simulink library "thermochemical"  (R2017b)
settings: Solver=VariableStepAuto  StartTime=0.0  StopTime=10.0  RelTol=1e-3
values from neighbouring files (symbols this model uses):
  c = conversion_factors()    [blk_clausius_clapeyron.m]    (also in blk_clausius_clapeyron_no_popup.m; blk_cold_room_closed_dry_air.m; blk_reactor_BaCl2_NH3_no_walls.m; blk_reactor_BaCl2_NH3_no_walls_state_space.m)
  cp = metal.cp    [blk_wall_simple.m]    (also in get_metal_properties.m = 390)
  fluid = get_param(blk,'fluid')    [blk_thermodynamic_properties_nonsaturated.m]    (also in blk_thermodynamic_properties_nonsaturated_interpreted.m; blk_thermodynamic_properties_saturated.m; blk_thermodynamic_properties_saturated_interpreted.m; blk_thermodynamic_properties_saturated_mix.m)
  gas = get_material_properties(x.gasName)    [blk_reactor_BaCl2_NH3_cylindrical_no_walls_fun1.m]
  h = get_param(gcb,'ObjectParameters')    [get_param_eval.m]
  rho = metal.rho    [blk_wall_simple.m]    (also in get_metal_properties.m = 8940)
  s = solve(eq,dx,'ReturnConditions',true)    [LMTD_inv.m]    (also in blk_wall_simple.m = get_param_eval(blk,'s'))
  u_gas_at_T_ref = -R * T_ref    [blk_reactor_BaCl2_NH3_no_walls.m]    (also in blk_reactor_BaCl2_NH3_no_walls_state_space.m)
undefined symbols (not defined in the file or in its folder): b_motor, BaCl2, beta, CoolProp, cP_binder, cP_gas, cP_s0, cv, dh_r_0, ENG, heat_exchanger_epsilonNTU_inv_simulink, heat_exchanger_epsilonNTU_simulink, J_motor, K_cin, kappa, Km_motor, La_motor, lookup2D_BreakPoint2, M_binder, N_binder, N_gas_free_volume_init, N_salt, NH3, nh3_v3, nu, P, phase, PID_D_motor, PID_I_motor, PID_P_motor, Ra_motor, Reactor_phase, T, T1, T2, T_init, Tr_init, Tr_ref, U_binder_at_Tr_ref, U_salt_at_X0_Tr_ref, Ur_init, V_void, Valve_regime, Vmax_motor, w_init_motor, X_init
libraries: thermochemical x247, simulink x54, dspsigops x3
(part 7 of 12)

== system thermochemical/Reactors/Reactor, BaCl2//NH3, state-space form, [Tr, Ng, X] as state variables, no algebraic loops, real gas in void volume, ideal gas in salt/Reactor, BaCl2, cylindrical, finned tube, state-space form, [Tr, Ng, X] as state variables, no algebraic loops, real gas in void volume, ideal gas in salt ==
  In3 : Inport
  In1 : Inport  Port=2
  In2 : Inport  Port=3
  In4 : Inport  Port=4
  Display4 : Display
  Gain : Gain  Gain=-1
  "Reactor, BaCl2/NH3, cylindrical, no walls, state-space form, [Tr, Ng, X] as state variables, no algebraic loops, real gas in void volume, ideal gas in salt" : thermochemical/Reactors/Reactor, BaCl2//NH3, state-space form, [Tr, Ng, X] as state variables, no algebraic loops, real gas in void volume, ideal gas in salt/Reactor, BaCl2//NH3, cylindrical, no walls, state-space form, [Tr, Ng, X] as state variables, no algebraic loops, real gas in void volume, ideal gas in salt  pairName=Barium chloride/Ammonia (BaCl2/NH3)  gasName=Ammonia gas (NH3)  binderName=ENG  tao_salt=0.75  rho_composite=300  K_cin=1e-3  fluid=nh3_v3  Lr=1.5  Lr_total=1.6  Dr=0.11  Ddiff=0.018  Tr_init=300  X_init=0.1  Vr_L=15.2053  m_composite_kg=4.162  m_salt_kg=3.1215  m_binder_kg=1.0405  m_gas_when_reactor_fully_charged_kg=2.0423  kWh_cold=0.77838  N_salt=14.9906  N_binder=86.6307  V_void=0.001332  N_gas_free_volume_init=0.16063
      settings: SourceProductName=@ Thermochemical
  "Wall, tube with/without fins" : thermochemical/Walls/Wall, tube with//without fins  L_m=1.6  OD_mm=114  e_mm=2  material_tube=Stainless steel AISI316  cp_tube=490.8  rho_tube=8023  height_fin_mm=0  thickness_fin_mm=0  pitch_fin_mm=0  material_fin=Steel  cp_fin=464.5  rho_fin=7847  lambda_fin=64.65  Tinit=300  mass_tube=4.5571  mass_fin=0  mass_total=4.5571  s_inner=0.56297  s_outer=0.57303
      settings: SourceProductName=@ Thermochemical
  composite-wall contact heat transfer coefficient (W/m2/K) : Constant  Value=300
  Out3 : Outport
  Out2 : Outport  Port=2
  Out4 : Outport  Port=3
  Out1 : Outport  Port=4
  Out5 : Outport  Port=5
  Out6 : Outport  Port=6
  Out7 : Outport  Port=7
  Out8 : Outport  Port=8
  wires:
  In4/1 -> "Reactor, BaCl2/NH3, cylindrical, no walls, state-space form, [Tr, Ng, X] as state variables, no algebraic loops, real gas in void volume, ideal gas in salt"/2  "enthalpy in (J/mol) (only needed if dn/dt gas > 0)"
  In2/1 -> "Reactor, BaCl2/NH3, cylindrical, no walls, state-space form, [Tr, Ng, X] as state variables, no algebraic loops, real gas in void volume, ideal gas in salt"/1  "dn/dt gas (mol/sec) > 0: gas in   < 0: gas out"
  "Wall, tube with/without fins"/1 -> Out3/1  "T wall (K)"
  "Reactor, BaCl2/NH3, cylindrical, no walls, state-space form, [Tr, Ng, X] as state variables, no algebraic loops, real gas in void volume, ideal gas in salt"/2 -> Out4/1  "Pr (bar)"
  "Reactor, BaCl2/NH3, cylindrical, no walls, state-space form, [Tr, Ng, X] as state variables, no algebraic loops, real gas in void volume, ideal gas in salt"/5 -> Out6/1  "X (0..1)"
  In1/1 -> "Wall, tube with/without fins"/2  "h outer (W/m2/K)"
  "Wall, tube with/without fins"/3 -> Out8/1  "Q wall → outer (W)"
  In3/1 -> "Wall, tube with/without fins"/1  "T outer (K)"
  "Reactor, BaCl2/NH3, cylindrical, no walls, state-space form, [Tr, Ng, X] as state variables, no algebraic loops, real gas in void volume, ideal gas in salt"/3 -> Out1/1  "h gas (void space) (J/mol)"
  composite-wall contact heat transfer coefficient (W/m2/K)/1 -> "Wall, tube with/without fins"/4
  "Wall, tube with/without fins"/2 -> Out7/1, Gain/1  "Q inner → wall (W)"
  "Reactor, BaCl2/NH3, cylindrical, no walls, state-space form, [Tr, Ng, X] as state variables, no algebraic loops, real gas in void volume, ideal gas in salt"/4 -> Out5/1  "Reaction phase"
  "Reactor, BaCl2/NH3, cylindrical, no walls, state-space form, [Tr, Ng, X] as state variables, no algebraic loops, real gas in void volume, ideal gas in salt"/1 -> "Wall, tube with/without fins"/3, Out2/1  "Tr (K)"
  "Wall, tube with/without fins"/4 -> Display4/1
  Gain/1 -> "Reactor, BaCl2/NH3, cylindrical, no walls, state-space form, [Tr, Ng, X] as state variables, no algebraic loops, real gas in void volume, ideal gas in salt"/3

== system thermochemical/Reactors/Reactor, BaCl2//NH3, state-space form, [Tr, Ng, X] as state variables, no algebraic loops, real gas in void volume, ideal gas in salt/Reactor, BaCl2//NH3, cylindrical, no walls, state-space form, [Tr, Ng, X] as state variables, no algebraic loops, real gas in void volume, ideal gas in salt ==
  In3 : Inport
  In2 : Inport  Port=2
  In4 : Inport  Port=3
  "Reactor, BaCl2/NH3, no walls, state-space form, [Tr, Ng, X] as state variables, no algebraic loops, real gas in void volume, ideal gas in salt" : thermochemical/Reactors/Reactor, BaCl2//NH3, state-space form, [Tr, Ng, X] as state variables, no algebraic loops, real gas in void volume, ideal gas in salt/Reactor, BaCl2//NH3, no walls, state-space form, [Tr, Ng, X] as state variables, no algebraic loops, real gas in void volume, ideal gas in salt  pairName=Barium chloride/Ammonia (BaCl2/NH3)  gasName=Ammonia gas (NH3)  binderName=ENG  N_salt=N_salt  N_binder=N_binder  K_cin=K_cin  V_void=V_void  fluid=fluid  Tr_init=Tr_init  X_init=X_init  N_gas_free_volume_init=N_gas_free_volume_init  m_composite_kg=4.1639  m_salt_kg=3.1235  m_binder_kg=1.0405  m_gas_when_reactor_fully_charged=2.0436  T_ref=300  u_gas_at_T_ref=0  U_binder_at_T_ref=0  U_salt_at_X0_T_ref=0  R=8.3145  cP_gas=42.5775  cV_gas=29.4370  nu=8  cP_s0=75.1  dh_r_0=38250  M_binder=0.012011  cP_binder=714.36  P_dead_zone=0.0001  dn_dead_zone=0.0001
      settings: SourceProductName=@ Thermochemical
  Out2 : Outport
  Out4 : Outport  Port=2
  Out3 : Outport  Port=3
  Out5 : Outport  Port=4
  Out1 : Outport  Port=5
  wires:
  In3/1 -> "Reactor, BaCl2/NH3, no walls, state-space form, [Tr, Ng, X] as state variables, no algebraic loops, real gas in void volume, ideal gas in salt"/1  "dn/dt gas (mol/sec) > 0: gas in   < 0: gas out"
  In2/1 -> "Reactor, BaCl2/NH3, no walls, state-space form, [Tr, Ng, X] as state variables, no algebraic loops, real gas in void volume, ideal gas in salt"/2  "enthalpy in (J/mol) (only needed if dn/dt gas > 0)"
  In4/1 -> "Reactor, BaCl2/NH3, no walls, state-space form, [Tr, Ng, X] as state variables, no algebraic loops, real gas in void volume, ideal gas in salt"/3  "q out → in (W)"
  "Reactor, BaCl2/NH3, no walls, state-space form, [Tr, Ng, X] as state variables, no algebraic loops, real gas in void volume, ideal gas in salt"/5 -> Out1/1  "X (0..1)"
  "Reactor, BaCl2/NH3, no walls, state-space form, [Tr, Ng, X] as state variables, no algebraic loops, real gas in void volume, ideal gas in salt"/4 -> Out5/1  "Reaction phase"
  "Reactor, BaCl2/NH3, no walls, state-space form, [Tr, Ng, X] as state variables, no algebraic loops, real gas in void volume, ideal gas in salt"/3 -> Out3/1  "h gas (void space) (J/mol)"
  "Reactor, BaCl2/NH3, no walls, state-space form, [Tr, Ng, X] as state variables, no algebraic loops, real gas in void volume, ideal gas in salt"/2 -> Out4/1  "Pr (bar)"
  "Reactor, BaCl2/NH3, no walls, state-space form, [Tr, Ng, X] as state variables, no algebraic loops, real gas in void volume, ideal gas in salt"/1 -> Out2/1  "Tr (K)"

== system thermochemical/Reactors/Reactor, BaCl2//NH3, state-space form, [Tr, Ng, X] as state variables, no algebraic loops, real gas in void volume, ideal gas in salt/Reactor, BaCl2//NH3, no walls, state-space form, [Tr, Ng, X] as state variables, no algebraic loops, real gas in void volume, ideal gas in salt ==
  In3 : Inport
  In2 : Inport  Port=2
  In4 : Inport  Port=3
  "Reactor, no walls, state space form" : Subsystem
  Out2 : Outport
  Out1 : Outport  Port=2
  Out5 : Outport  Port=3
  Out3 : Outport  Port=4
  Out4 : Outport  Port=5
  wires:
  In3/1 -> "Reactor, no walls, state space form"/2(enthalpy_in (J/mol) (only if dn_gas > 0))  "dn/dt gas (mol/sec) > 0: gas in   < 0: gas out"
  In2/1 -> "Reactor, no walls, state space form"/3(In3)  "enthalpy in (J/mol) (only needed if dn/dt gas > 0)"
  In4/1 -> "Reactor, no walls, state space form"/1(q reactor → wall (W))  "q out → in (W)"
  "Reactor, no walls, state space form"/2(Reactor phase) -> Out1/1  "Pr (bar)"
  "Reactor, no walls, state space form"/4(T_reactor (K)) -> Out5/1  "h gas void space (J/mol)"
  "Reactor, no walls, state space form"/5(h_reactor_free_volume (J/mol)) -> Out3/1  "Reaction phase"
  "Reactor, no walls, state space form"/3(P_reactor (bar)) -> Out4/1  "X (0..1)"
  "Reactor, no walls, state space form"/1(X (0..1)) -> Out2/1  "Tr (K)"

== system thermochemical/Reactors/Reactor, BaCl2//NH3, state-space form, [Tr, Ng, X] as state variables, no algebraic loops, real gas in void volume, real gas in salt/Reactor, BaCl2, cylindrical, finned tube, state-space form, [Tr, Ng, X] as state variables, no algebraic loops, real gas in void volume, real gas in salt ==
  In3 : Inport
  In1 : Inport  Port=2
  In2 : Inport  Port=3
  In4 : Inport  Port=4
  Display4 : Display
  Gain : Gain  Gain=-1
  "Reactor, BaCl2/NH3, cylindrical, no walls, state-space form, [Tr, Ng, X] as state variables, no algebraic loops, real gas in void volume, real gas in salt" : thermochemical/Reactors/Reactor, BaCl2//NH3, state-space form, [Tr, Ng, X] as state variables, no algebraic loops, real gas in void volume, real gas in salt/Reactor, BaCl2//NH3, cylindrical, no walls, state-space form, [Tr, Ng, X] as state variables, no algebraic loops, real gas in void volume, real gas in salt  pairName=Barium chloride/Ammonia (BaCl2/NH3)  gasName=Ammonia gas (NH3)  binderName=ENG  tao_salt=0.75  rho_composite=300  K_cin=1e-3  fluid=nh3_v3  Lr=1.5  Lr_total=1.6  Dr=0.11  Ddiff=0.018  Tr_init=300  X_init=0.1  Vr_L=15.2053  m_composite_kg=4.162  m_salt_kg=3.1215  m_binder_kg=1.0405  m_gas_when_reactor_fully_charged_kg=2.0423  kWh_cold=0.77838  N_salt=14.9906  N_binder=86.6307  V_void=0.001332  N_gas_free_volume_init=0.16063
      settings: SourceProductName=@ Thermochemical
  "Wall, tube with/without fins" : thermochemical/Walls/Wall, tube with//without fins  L_m=1.6  OD_mm=114  e_mm=2  material_tube=Stainless steel AISI316  cp_tube=490.8  rho_tube=8023  height_fin_mm=0  thickness_fin_mm=0  pitch_fin_mm=0  material_fin=Steel  cp_fin=464.5  rho_fin=7847  lambda_fin=64.65  Tinit=300  mass_tube=9.0335  mass_fin=0  mass_total=9.0335  s_inner=0.55292  s_outer=0.57303
      settings: SourceProductName=@ Thermochemical
  composite-wall contact heat transfer coefficient (W/m2/K) : Constant  Value=300
  Out3 : Outport
  Out2 : Outport  Port=2
  Out4 : Outport  Port=3
  Out1 : Outport  Port=4
  Out5 : Outport  Port=5
  Out6 : Outport  Port=6
  Out7 : Outport  Port=7
  Out8 : Outport  Port=8
  wires:
  In4/1 -> "Reactor, BaCl2/NH3, cylindrical, no walls, state-space form, [Tr, Ng, X] as state variables, no algebraic loops, real gas in void volume, real gas in salt"/2  "enthalpy in (J/mol) (only needed if dn/dt gas > 0)"
  In2/1 -> "Reactor, BaCl2/NH3, cylindrical, no walls, state-space form, [Tr, Ng, X] as state variables, no algebraic loops, real gas in void volume, real gas in salt"/1  "dn/dt gas (mol/sec) > 0: gas in   < 0: gas out"
  "Wall, tube with/without fins"/1 -> Out3/1  "T wall (K)"
  "Reactor, BaCl2/NH3, cylindrical, no walls, state-space form, [Tr, Ng, X] as state variables, no algebraic loops, real gas in void volume, real gas in salt"/2 -> Out4/1  "Pr (bar)"
  "Reactor, BaCl2/NH3, cylindrical, no walls, state-space form, [Tr, Ng, X] as state variables, no algebraic loops, real gas in void volume, real gas in salt"/5 -> Out6/1  "X (0..1)"
  In1/1 -> "Wall, tube with/without fins"/2  "h outer (W/m2/K)"
  "Wall, tube with/without fins"/3 -> Out8/1  "Q wall → outer (W)"
  In3/1 -> "Wall, tube with/without fins"/1  "T outer (K)"
  "Reactor, BaCl2/NH3, cylindrical, no walls, state-space form, [Tr, Ng, X] as state variables, no algebraic loops, real gas in void volume, real gas in salt"/3 -> Out1/1  "h gas (void space) (J/mol)"
  composite-wall contact heat transfer coefficient (W/m2/K)/1 -> "Wall, tube with/without fins"/4
  "Wall, tube with/without fins"/2 -> Out7/1, Gain/1  "Q inner → wall (W)"
  "Reactor, BaCl2/NH3, cylindrical, no walls, state-space form, [Tr, Ng, X] as state variables, no algebraic loops, real gas in void volume, real gas in salt"/4 -> Out5/1  "Reaction phase"
  "Reactor, BaCl2/NH3, cylindrical, no walls, state-space form, [Tr, Ng, X] as state variables, no algebraic loops, real gas in void volume, real gas in salt"/1 -> "Wall, tube with/without fins"/3, Out2/1  "Tr (K)"
  "Wall, tube with/without fins"/4 -> Display4/1
  Gain/1 -> "Reactor, BaCl2/NH3, cylindrical, no walls, state-space form, [Tr, Ng, X] as state variables, no algebraic loops, real gas in void volume, real gas in salt"/3

== system thermochemical/Reactors/Reactor, BaCl2//NH3, state-space form, [Tr, Ng, X] as state variables, no algebraic loops, real gas in void volume, real gas in salt/Reactor, BaCl2//NH3, cylindrical, no walls, state-space form, [Tr, Ng, X] as state variables, no algebraic loops, real gas in void volume, real gas in salt ==
  In3 : Inport
  In2 : Inport  Port=2
  In4 : Inport  Port=3
  "Reactor, BaCl2/NH3, no walls, state-space form, [Tr, Ng, X] as state variables, no algebraic loops, real gas in void volume, real gas in salt" : thermochemical/Reactors/Reactor, BaCl2//NH3, state-space form, [Tr, Ng, X] as state variables, no algebraic loops, real gas in void volume, real gas in salt/Reactor, BaCl2//NH3, no walls, state-space form, [Tr, Ng, X] as state variables, no algebraic loops, real gas in void volume, real gas in salt  pairName=Barium chloride/Ammonia (BaCl2/NH3)  gasName=Ammonia gas (NH3)  binderName=ENG  N_salt=N_salt  N_binder=N_binder  K_cin=K_cin  V_void=V_void  fluid=fluid  Tr_init=Tr_init  X_init=X_init  N_gas_free_volume_init=N_gas_free_volume_init  m_composite_kg=4.1639  m_salt_kg=3.1235  m_binder_kg=1.0405  m_gas_when_reactor_fully_charged=2.0436  T_ref=300  u_gas_at_T_ref=0  U_binder_at_T_ref=0  U_salt_at_X0_T_ref=0  R=8.3145  cP_gas=42.5775  cV_gas=29.4370  nu=8  cP_s0=75.1  dh_r_0=38250  M_binder=0.012011  cP_binder=714.36  P_dead_zone=0.0001  dn_dead_zone=0.0001
      settings: SourceProductName=@ Thermochemical
  Out2 : Outport
  Out4 : Outport  Port=2
  Out3 : Outport  Port=3
  Out5 : Outport  Port=4
  Out1 : Outport  Port=5
  wires:
  In3/1 -> "Reactor, BaCl2/NH3, no walls, state-space form, [Tr, Ng, X] as state variables, no algebraic loops, real gas in void volume, real gas in salt"/1  "dn/dt gas (mol/sec) > 0: gas in   < 0: gas out"
  In2/1 -> "Reactor, BaCl2/NH3, no walls, state-space form, [Tr, Ng, X] as state variables, no algebraic loops, real gas in void volume, real gas in salt"/2  "enthalpy in (J/mol) (only needed if dn/dt gas > 0)"
  In4/1 -> "Reactor, BaCl2/NH3, no walls, state-space form, [Tr, Ng, X] as state variables, no algebraic loops, real gas in void volume, real gas in salt"/3  "q out → in (W)"
  "Reactor, BaCl2/NH3, no walls, state-space form, [Tr, Ng, X] as state variables, no algebraic loops, real gas in void volume, real gas in salt"/5 -> Out1/1  "X (0..1)"
  "Reactor, BaCl2/NH3, no walls, state-space form, [Tr, Ng, X] as state variables, no algebraic loops, real gas in void volume, real gas in salt"/4 -> Out5/1  "Reaction phase"
  "Reactor, BaCl2/NH3, no walls, state-space form, [Tr, Ng, X] as state variables, no algebraic loops, real gas in void volume, real gas in salt"/3 -> Out3/1  "h gas (void space) (J/mol)"
  "Reactor, BaCl2/NH3, no walls, state-space form, [Tr, Ng, X] as state variables, no algebraic loops, real gas in void volume, real gas in salt"/2 -> Out4/1  "Pr (bar)"
  "Reactor, BaCl2/NH3, no walls, state-space form, [Tr, Ng, X] as state variables, no algebraic loops, real gas in void volume, real gas in salt"/1 -> Out2/1  "Tr (K)"

== system thermochemical/Reactors/Reactor, BaCl2//NH3, state-space form, [Tr, Ng, X] as state variables, no algebraic loops, real gas in void volume, real gas in salt/Reactor, BaCl2//NH3, no walls, state-space form, [Tr, Ng, X] as state variables, no algebraic loops, real gas in void volume, real gas in salt ==
  In3 : Inport
  In2 : Inport  Port=2
  In4 : Inport  Port=3
  "Reactor, no walls, state space form" : Subsystem
  Out2 : Outport
  Out1 : Outport  Port=2
  Out5 : Outport  Port=3
  Out3 : Outport  Port=4
  Out4 : Outport  Port=5
  wires:
  "Reactor, no walls, state space form"/1(X (0..1)) -> Out2/1  "Tr (K)"
  "Reactor, no walls, state space form"/3(P_reactor (bar)) -> Out4/1  "X (0..1)"
  "Reactor, no walls, state space form"/5(h_reactor_free_volume (J/mol)) -> Out3/1  "Reaction phase"
  "Reactor, no walls, state space form"/4(T_reactor (K)) -> Out5/1  "h gas void space (J/mol)"
  "Reactor, no walls, state space form"/2(Reactor phase) -> Out1/1  "Pr (bar)"
  In4/1 -> "Reactor, no walls, state space form"/1(q reactor → wall (W))  "q out → in (W)"
  In2/1 -> "Reactor, no walls, state space form"/3(In3)  "enthalpy in (J/mol) (only needed if dn/dt gas > 0)"
  In3/1 -> "Reactor, no walls, state space form"/2(enthalpy_in (J/mol) (only if dn_gas > 0))  "dn/dt gas (mol/sec) > 0: gas in   < 0: gas out"

== system thermochemical/Reactors/Reactor, BaCl2//NH3, state-space form, [Ur, Ng, X] as state variables, no algebraic loops, ideal gas in void volume, ideal gas in salt/Reactor, BaCl2, cylindrical, finned tube, state-space form, [Ur, Ng, X] as state variables, no algebraic loops, ideal gas in void volume, ideal gas in salt ==
  In3 : Inport
  In1 : Inport  Port=2
  In2 : Inport  Port=3
  In4 : Inport  Port=4
  Display4 : Display
  Gain : Gain  Gain=-1
  "Reactor, BaCl2/NH3, cylindrical, no walls, state-space form, [Ur, Ng, X] as state variables, no algebraic loops, ideal gas in void volume, ideal gas in salt" : thermochemical/Reactors/Reactor, BaCl2//NH3, state-space form, [Ur, Ng, X] as state variables, no algebraic loops, ideal gas in void volume, ideal gas in salt/Reactor, BaCl2//NH3, cylindrical, no walls, state-space form, [Ur, Ng, X] as state variables, no algebraic loops, ideal gas in void volume, ideal gas in salt  pairName=Barium chloride/Ammonia (BaCl2/NH3)  gasName=Ammonia gas (NH3)  binderName=ENG  tao_salt=0.75  rho_composite=300  K_cin=1e-3  fluid=nh3_v3  Lr=1.5  Lr_total=1.6  Dr=0.11  Ddiff=0.018  Tr_init=300  X_init=0.1  Vr_L=15.2053  m_composite_kg=4.162  m_salt_kg=3.1215  m_binder_kg=1.0405  m_gas_when_reactor_fully_charged_kg=2.0423  kWh_cold=0.77838  N_salt=14.9906  N_binder=86.6307  V_void=0.001332  N_gas_free_volume_init=0.16063
      settings: SourceProductName=@ Thermochemical
  "Wall, tube with/without fins" : thermochemical/Walls/Wall, tube with//without fins  L_m=1.6  OD_mm=114  e_mm=2  material_tube=Stainless steel AISI316  cp_tube=490.8  rho_tube=8023  height_fin_mm=0  thickness_fin_mm=0  pitch_fin_mm=0  material_fin=Steel  cp_fin=464.5  rho_fin=7847  lambda_fin=64.65  Tinit=300  mass_tube=4.5571  mass_fin=0  mass_total=4.5571  s_inner=0.56297  s_outer=0.57303
      settings: SourceProductName=@ Thermochemical
  composite-wall contact heat transfer coefficient (W/m2/K) : Constant  Value=300
  Out3 : Outport
  Out2 : Outport  Port=2
  Out4 : Outport  Port=3
  Out1 : Outport  Port=4
  Out5 : Outport  Port=5
  Out6 : Outport  Port=6
  Out7 : Outport  Port=7
  Out8 : Outport  Port=8
  wires:
  In4/1 -> "Reactor, BaCl2/NH3, cylindrical, no walls, state-space form, [Ur, Ng, X] as state variables, no algebraic loops, ideal gas in void volume, ideal gas in salt"/2  "enthalpy in (J/mol) (only needed if dn/dt gas > 0)"
  In2/1 -> "Reactor, BaCl2/NH3, cylindrical, no walls, state-space form, [Ur, Ng, X] as state variables, no algebraic loops, ideal gas in void volume, ideal gas in salt"/1  "dn/dt gas (mol/sec) > 0: gas in   < 0: gas out"
  "Wall, tube with/without fins"/1 -> Out3/1  "T wall (K)"
  "Reactor, BaCl2/NH3, cylindrical, no walls, state-space form, [Ur, Ng, X] as state variables, no algebraic loops, ideal gas in void volume, ideal gas in salt"/2 -> Out4/1  "Pr (bar)"
  "Reactor, BaCl2/NH3, cylindrical, no walls, state-space form, [Ur, Ng, X] as state variables, no algebraic loops, ideal gas in void volume, ideal gas in salt"/5 -> Out6/1  "X (0..1)"
  In1/1 -> "Wall, tube with/without fins"/2  "h outer (W/m2/K)"
  "Wall, tube with/without fins"/3 -> Out8/1  "Q wall → outer (W)"
  In3/1 -> "Wall, tube with/without fins"/1  "T outer (K)"
  "Reactor, BaCl2/NH3, cylindrical, no walls, state-space form, [Ur, Ng, X] as state variables, no algebraic loops, ideal gas in void volume, ideal gas in salt"/3 -> Out1/1  "h gas (void space) (J/mol)"
  composite-wall contact heat transfer coefficient (W/m2/K)/1 -> "Wall, tube with/without fins"/4
  "Wall, tube with/without fins"/2 -> Out7/1, Gain/1  "Q inner → wall (W)"
  "Reactor, BaCl2/NH3, cylindrical, no walls, state-space form, [Ur, Ng, X] as state variables, no algebraic loops, ideal gas in void volume, ideal gas in salt"/4 -> Out5/1  "Reaction phase"
  "Reactor, BaCl2/NH3, cylindrical, no walls, state-space form, [Ur, Ng, X] as state variables, no algebraic loops, ideal gas in void volume, ideal gas in salt"/1 -> "Wall, tube with/without fins"/3, Out2/1  "Tr (K)"
  "Wall, tube with/without fins"/4 -> Display4/1
  Gain/1 -> "Reactor, BaCl2/NH3, cylindrical, no walls, state-space form, [Ur, Ng, X] as state variables, no algebraic loops, ideal gas in void volume, ideal gas in salt"/3

== system thermochemical/Reactors/Reactor, BaCl2//NH3, state-space form, [Ur, Ng, X] as state variables, no algebraic loops, ideal gas in void volume, ideal gas in salt/Reactor, BaCl2//NH3, cylindrical, no walls, state-space form, [Ur, Ng, X] as state variables, no algebraic loops, ideal gas in void volume, ideal gas in salt ==
  In3 : Inport
  In2 : Inport  Port=2
  In4 : Inport  Port=3
  "Reactor, BaCl2/NH3, no walls, state-space form, [Ur, Ng, X] as state variables, no algebraic loops, ideal gas in void volume, ideal gas in salt" : thermochemical/Reactors/Reactor, BaCl2//NH3, state-space form, [Ur, Ng, X] as state variables, no algebraic loops, ideal gas in void volume, ideal gas in salt/Reactor, BaCl2//NH3, no walls, state-space form, [Ur, Ng, X] as state variables, no algebraic loops, ideal gas in void volume, ideal gas in salt  pairName=Barium chloride/Ammonia (BaCl2/NH3)  gasName=Ammonia gas (NH3)  binderName=ENG  N_salt=N_salt  N_binder=N_binder  K_cin=K_cin  V_void=V_void  Tr_init=Tr_init  X_init=X_init  N_gas_free_volume_init=N_gas_free_volume_init  T_ref=239.8236  u_gas_at_T_ref=-1994.0066  U_binder_at_T_ref=0  U_salt_at_X0_T_ref=0  R=8.3145  cP_gas=42.5775  nu=8  cP_s0=75.1  dh_r_0=38250  M_binder=0.012011  cP_binder=714.36  P_dead_zone=0.0001  dn_dead_zone=0.0001
      settings: SourceProductName=@ Thermochemical
  Out2 : Outport
  Out4 : Outport  Port=2
  Out3 : Outport  Port=3
  Out5 : Outport  Port=4
  Out1 : Outport  Port=5
  wires:
  In3/1 -> "Reactor, BaCl2/NH3, no walls, state-space form, [Ur, Ng, X] as state variables, no algebraic loops, ideal gas in void volume, ideal gas in salt"/1  "dn/dt gas (mol/sec) > 0: gas in   < 0: gas out"
  In2/1 -> "Reactor, BaCl2/NH3, no walls, state-space form, [Ur, Ng, X] as state variables, no algebraic loops, ideal gas in void volume, ideal gas in salt"/2  "enthalpy in (J/mol) (only needed if dn/dt gas > 0)"
  In4/1 -> "Reactor, BaCl2/NH3, no walls, state-space form, [Ur, Ng, X] as state variables, no algebraic loops, ideal gas in void volume, ideal gas in salt"/3  "q out → in (W)"
  "Reactor, BaCl2/NH3, no walls, state-space form, [Ur, Ng, X] as state variables, no algebraic loops, ideal gas in void volume, ideal gas in salt"/5 -> Out1/1  "X (0..1)"
  "Reactor, BaCl2/NH3, no walls, state-space form, [Ur, Ng, X] as state variables, no algebraic loops, ideal gas in void volume, ideal gas in salt"/4 -> Out5/1  "Reaction phase"
  "Reactor, BaCl2/NH3, no walls, state-space form, [Ur, Ng, X] as state variables, no algebraic loops, ideal gas in void volume, ideal gas in salt"/3 -> Out3/1  "h gas (void space) (J/mol)"
  "Reactor, BaCl2/NH3, no walls, state-space form, [Ur, Ng, X] as state variables, no algebraic loops, ideal gas in void volume, ideal gas in salt"/2 -> Out4/1  "Pr (bar)"
  "Reactor, BaCl2/NH3, no walls, state-space form, [Ur, Ng, X] as state variables, no algebraic loops, ideal gas in void volume, ideal gas in salt"/1 -> Out2/1  "Tr (K)"

== system thermochemical/Reactors/Reactor, BaCl2//NH3, state-space form, [Ur, Ng, X] as state variables, no algebraic loops, ideal gas in void volume, ideal gas in salt/Reactor, BaCl2//NH3, no walls, state-space form, [Ur, Ng, X] as state variables, no algebraic loops, ideal gas in void volume, ideal gas in salt ==
  In3 : Inport
  In2 : Inport  Port=2
  In4 : Inport  Port=3
  "Reactor, no walls, state space form" : Subsystem
  Out2 : Outport
  Out1 : Outport  Port=2
  Out5 : Outport  Port=3
  Out3 : Outport  Port=4
  Out4 : Outport  Port=5
  wires:
  "Reactor, no walls, state space form"/1(X (0..1)) -> Out2/1  "Tr (K)"
  "Reactor, no walls, state space form"/3(P_reactor (bar)) -> Out4/1  "X (0..1)"
  "Reactor, no walls, state space form"/5(h_reactor_free_volume (J/mol)) -> Out3/1  "Reaction phase"
  "Reactor, no walls, state space form"/4(T_reactor (K)) -> Out5/1  "h gas void space (J/mol)"
  "Reactor, no walls, state space form"/2(Reactor phase) -> Out1/1  "Pr (bar)"
  In4/1 -> "Reactor, no walls, state space form"/1(q reactor → wall (W))  "q out → in (W)"
  In2/1 -> "Reactor, no walls, state space form"/3(In3)  "enthalpy in (J/mol) (only needed if dn/dt gas > 0)"
  In3/1 -> "Reactor, no walls, state space form"/2(enthalpy_in (J/mol) (only if dn_gas > 0))  "dn/dt gas (mol/sec) > 0: gas in   < 0: gas out"

== system thermochemical/Reactors/Reactor, BaCl2//NH3, with algebraic loops, ideal gas in void volume, ideal gas in salt/Reactor, BaCl2, cylindrical, finned tube, with algebraic loops, ideal gas in void volume, ideal gas in salt ==
  In3 : Inport
  In1 : Inport  Port=2
  In2 : Inport  Port=3
  In4 : Inport  Port=4
  Display4 : Display
  Gain : Gain  Gain=-1
  "Reactor, BaCl2/NH3, cylindrical, no walls, with algebraic loops, ideal gas in void volume, ideal gas in salt" : thermochemical/Reactors/Reactor, BaCl2//NH3, with algebraic loops, ideal gas in void volume, ideal gas in salt/Reactor, BaCl2//NH3, cylindrical, no walls, with algebraic loops, ideal gas in void volume, ideal gas in salt  pairName=Barium chloride/Ammonia (BaCl2/NH3)  gasName=Ammonia gas (NH3)  binderName=ENG  tao_salt=0.75  rho_composite=300  K_cin=1e-3  fluid=nh3_v3  Lr=1.5  Lr_total=1.6  Dr=0.11  Ddiff=0.018  Tr_init=300  X_init=0.1  Vr_L=15.2053  m_composite_kg=4.162  m_salt_kg=3.1215  m_binder_kg=1.0405  m_gas_when_reactor_fully_charged_kg=2.0423  kWh_cold=0.77838  N_salt=14.9906  N_binder=86.6307  V_void=0.001332  N_gas_free_volume_init=0.16063
      settings: SourceProductName=@ Thermochemical
  "Wall, tube with/without fins" : thermochemical/Walls/Wall, tube with//without fins  L_m=1.6  OD_mm=114  e_mm=2  material_tube=Stainless steel AISI316  cp_tube=490.8  rho_tube=8023  height_fin_mm=0  thickness_fin_mm=0  pitch_fin_mm=0  material_fin=Steel  cp_fin=464.5  rho_fin=7847  lambda_fin=64.65  Tinit=300  mass_tube=4.5571  mass_fin=0  mass_total=4.5571  s_inner=0.56297  s_outer=0.57303
      settings: SourceProductName=@ Thermochemical
  composite-wall contact heat transfer coefficient (W/m2/K) : Constant  Value=300
  Out3 : Outport
  Out2 : Outport  Port=2
  Out4 : Outport  Port=3
  Out1 : Outport  Port=4
  Out5 : Outport  Port=5
  Out6 : Outport  Port=6
  Out7 : Outport  Port=7
  Out8 : Outport  Port=8
  wires:
  Gain/1 -> "Reactor, BaCl2/NH3, cylindrical, no walls, with algebraic loops, ideal gas in void volume, ideal gas in salt"/3
  "Wall, tube with/without fins"/4 -> Display4/1
  "Reactor, BaCl2/NH3, cylindrical, no walls, with algebraic loops, ideal gas in void volume, ideal gas in salt"/1 -> Out2/1, "Wall, tube with/without fins"/3  "Tr (K)"
  "Reactor, BaCl2/NH3, cylindrical, no walls, with algebraic loops, ideal gas in void volume, ideal gas in salt"/4 -> Out5/1  "Reaction phase"
  "Wall, tube with/without fins"/2 -> Gain/1, Out7/1  "Q inner → wall (W)"
  composite-wall contact heat transfer coefficient (W/m2/K)/1 -> "Wall, tube with/without fins"/4
  "Reactor, BaCl2/NH3, cylindrical, no walls, with algebraic loops, ideal gas in void volume, ideal gas in salt"/3 -> Out1/1  "h gas (void space) (J/mol)"
  In3/1 -> "Wall, tube with/without fins"/1  "T outer (K)"
  "Wall, tube with/without fins"/3 -> Out8/1  "Q wall → outer (W)"
  In1/1 -> "Wall, tube with/without fins"/2  "h outer (W/m2/K)"
  "Reactor, BaCl2/NH3, cylindrical, no walls, with algebraic loops, ideal gas in void volume, ideal gas in salt"/5 -> Out6/1  "X (0..1)"
  "Reactor, BaCl2/NH3, cylindrical, no walls, with algebraic loops, ideal gas in void volume, ideal gas in salt"/2 -> Out4/1  "Pr (bar)"
  "Wall, tube with/without fins"/1 -> Out3/1  "T wall (K)"
  In2/1 -> "Reactor, BaCl2/NH3, cylindrical, no walls, with algebraic loops, ideal gas in void volume, ideal gas in salt"/1  "dn/dt gas (mol/sec) > 0: gas in   < 0: gas out"
  In4/1 -> "Reactor, BaCl2/NH3, cylindrical, no walls, with algebraic loops, ideal gas in void volume, ideal gas in salt"/2  "enthalpy in (J/mol) (only needed if dn/dt gas > 0)"

== system thermochemical/Reactors/Reactor, BaCl2//NH3, with algebraic loops, ideal gas in void volume, ideal gas in salt/Reactor, BaCl2//NH3, cylindrical, no walls, with algebraic loops, ideal gas in void volume, ideal gas in salt ==
  In3 : Inport
  In2 : Inport  Port=2
  In4 : Inport  Port=3
  "Reactor, BaCl2/NH3, no walls, with algebraic loops, ideal gas in void volume, ideal gas in salt" : thermochemical/Reactors/Reactor, BaCl2//NH3, with algebraic loops, ideal gas in void volume, ideal gas in salt/Reactor, BaCl2//NH3, no walls, with algebraic loops, ideal gas in void volume, ideal gas in salt  pairName=Barium chloride/Ammonia (BaCl2/NH3)  gasName=Ammonia gas (NH3)  binderName=ENG  N_salt=N_salt  N_binder=N_binder  K_cin=K_cin  V_void=V_void  fluid=fluid  Tr_init=Tr_init  X_init=X_init  N_gas_free_volume_init=N_gas_free_volume_init  m_composite_kg=4.162  m_salt_kg=3.1215  m_binder_kg=1.0405  m_gas_when_reactor_fully_charged=2.0424  T_ref=239.8236  u_gas_at_T_ref=-1994.0066  U_binder_at_T_ref=0  U_salt_at_X0_T_ref=0  cP_gas=42.5775  nu=8  cP_s0=75.1  Pr_0=1e-05  dh_r_0=38250  ds_r_0=232.38  M_binder=0.012011  cP_binder=714.36  P_dead_zone=0.0001  dn_dead_zone=0.0001  R=8.3145
      settings: SourceProductName=@ Thermochemical
  Out2 : Outport
  Out4 : Outport  Port=2
  Out3 : Outport  Port=3
  Out5 : Outport  Port=4
  Out1 : Outport  Port=5
  wires:
  "Reactor, BaCl2/NH3, no walls, with algebraic loops, ideal gas in void volume, ideal gas in salt"/1 -> Out2/1  "Tr (K)"
  "Reactor, BaCl2/NH3, no walls, with algebraic loops, ideal gas in void volume, ideal gas in salt"/2 -> Out4/1  "Pr (bar)"
  "Reactor, BaCl2/NH3, no walls, with algebraic loops, ideal gas in void volume, ideal gas in salt"/3 -> Out3/1  "h gas (void space) (J/mol)"
  "Reactor, BaCl2/NH3, no walls, with algebraic loops, ideal gas in void volume, ideal gas in salt"/4 -> Out5/1  "Reaction phase"
  "Reactor, BaCl2/NH3, no walls, with algebraic loops, ideal gas in void volume, ideal gas in salt"/5 -> Out1/1  "X (0..1)"
  In4/1 -> "Reactor, BaCl2/NH3, no walls, with algebraic loops, ideal gas in void volume, ideal gas in salt"/3  "q out → in (W)"
  In2/1 -> "Reactor, BaCl2/NH3, no walls, with algebraic loops, ideal gas in void volume, ideal gas in salt"/2  "enthalpy in (J/mol) (only needed if dn/dt gas > 0)"
  In3/1 -> "Reactor, BaCl2/NH3, no walls, with algebraic loops, ideal gas in void volume, ideal gas in salt"/1  "dn/dt gas (mol/sec) > 0: gas in   < 0: gas out"

== system thermochemical/Reactors/Reactor, BaCl2//NH3, with algebraic loops, ideal gas in void volume, ideal gas in salt/Reactor, BaCl2//NH3, no walls, with algebraic loops, ideal gas in void volume, ideal gas in salt ==
  In3 : Inport
  In2 : Inport  Port=2
  In4 : Inport  Port=3
  Reactor (no walls) : Subsystem
  Out2 : Outport
  Out1 : Outport  Port=2
  Out5 : Outport  Port=3
  Out3 : Outport  Port=4
  Out4 : Outport  Port=5
  wires:
  Reactor (no walls)/5(P_reactor (bar)) -> Out1/1  "Pr (bar)"
  Reactor (no walls)/4(h_reactor_free_volume (J/mol)) -> Out5/1  "h gas void space (J/mol)"
  Reactor (no walls)/3(Reactor phase) -> Out3/1  "Reaction phase"
  Reactor (no walls)/2(X (0..1)) -> Out4/1  "X (0..1)"
  In3/1 -> Reactor (no walls)/3(dn_gas (mol/sec) (if > 0: gas in if < 0: gas out))  "dn/dt gas (mol/sec) > 0: gas in   < 0: gas out"
  In2/1 -> Reactor (no walls)/2(enthalpy_in (J/mol) (only if dn_gas > 0))  "enthalpy in (J/mol) (only needed if dn/dt gas > 0)"
  In4/1 -> Reactor (no walls)/1(q reactor → wall (W))  "q out → in (W)"
  Reactor (no walls)/1(T_reactor (K)) -> Out2/1  "Tr (K)"

== system thermochemical/Reactors/Reactor, BaCl2//NH3, with algebraic loops, real gas in void volume, ideal gas in salt/Reactor, BaCl2//NH3, cylindrical, finned tube, with algebraic loops, real gas in void volume, ideal gas in salt ==
  In3 : Inport
  In1 : Inport  Port=2
  In2 : Inport  Port=3
  In4 : Inport  Port=4
  Display4 : Display
  Gain : Gain  Gain=-1
  "Reactor, BaCl2/NH3, cylindrical, no walls, with algebraic loops, real gas in void volume, ideal gas in salt" : thermochemical/Reactors/Reactor, BaCl2//NH3, with algebraic loops, real gas in void volume, ideal gas in salt/Reactor, BaCl2//NH3, cylindrical, no walls, with algebraic loops, real gas in void volume, ideal gas in salt  pairName=Barium chloride/Ammonia (BaCl2/NH3)  gasName=Ammonia gas (NH3)  binderName=ENG  tao_salt=0.75  rho_composite=300  K_cin=1e-3  fluid=nh3_v3  Lr=1.5  Lr_total=1.6  Dr=0.11  Ddiff=0.018  Tr_init=300  X_init=0.1  Vr_L=15.2053  m_composite_kg=4.162  m_salt_kg=3.1215  m_binder_kg=1.0405  m_gas_when_reactor_fully_charged_kg=2.0423  kWh_cold=0.77838  N_salt=14.9906  N_binder=86.6307  V_void=0.001332  N_gas_free_volume_init=0.16063
      settings: SourceProductName=@ Thermochemical
  "Wall, tube with/without fins" : thermochemical/Walls/Wall, tube with//without fins  L_m=1.6  OD_mm=114  e_mm=2  material_tube=Stainless steel AISI316  cp_tube=490.8  rho_tube=8023  height_fin_mm=0  thickness_fin_mm=0  pitch_fin_mm=0  material_fin=Steel  cp_fin=464.5  rho_fin=7847  lambda_fin=64.65  Tinit=300  mass_tube=9.0335  mass_fin=0  mass_total=9.0335  s_inner=0.55292  s_outer=0.57303
      settings: SourceProductName=@ Thermochemical
  composite-wall contact heat transfer coefficient (W/m2/K) : Constant  Value=300
  Out3 : Outport
  Out2 : Outport  Port=2
  Out4 : Outport  Port=3
  Out1 : Outport  Port=4
  Out5 : Outport  Port=5
  Out6 : Outport  Port=6
  Out7 : Outport  Port=7
  Out8 : Outport  Port=8
  wires:
  In4/1 -> "Reactor, BaCl2/NH3, cylindrical, no walls, with algebraic loops, real gas in void volume, ideal gas in salt"/2  "enthalpy in (J/mol) (only needed if dn/dt gas > 0)"
  In2/1 -> "Reactor, BaCl2/NH3, cylindrical, no walls, with algebraic loops, real gas in void volume, ideal gas in salt"/1  "dn/dt gas (mol/sec) > 0: gas in   < 0: gas out"
  "Wall, tube with/without fins"/1 -> Out3/1  "T wall (K)"
  "Reactor, BaCl2/NH3, cylindrical, no walls, with algebraic loops, real gas in void volume, ideal gas in salt"/2 -> Out4/1  "Pr (bar)"
  "Reactor, BaCl2/NH3, cylindrical, no walls, with algebraic loops, real gas in void volume, ideal gas in salt"/5 -> Out6/1  "X (0..1)"
  In1/1 -> "Wall, tube with/without fins"/2  "h outer (W/m2/K)"
  "Wall, tube with/without fins"/3 -> Out8/1  "Q wall → outer (W)"
  In3/1 -> "Wall, tube with/without fins"/1  "T outer (K)"
  "Reactor, BaCl2/NH3, cylindrical, no walls, with algebraic loops, real gas in void volume, ideal gas in salt"/3 -> Out1/1  "h gas (void space) (J/mol)"
  composite-wall contact heat transfer coefficient (W/m2/K)/1 -> "Wall, tube with/without fins"/4
  "Wall, tube with/without fins"/2 -> Out7/1, Gain/1  "Q inner → wall (W)"
  "Reactor, BaCl2/NH3, cylindrical, no walls, with algebraic loops, real gas in void volume, ideal gas in salt"/4 -> Out5/1  "Reaction phase"
  "Reactor, BaCl2/NH3, cylindrical, no walls, with algebraic loops, real gas in void volume, ideal gas in salt"/1 -> "Wall, tube with/without fins"/3, Out2/1  "Tr (K)"
  "Wall, tube with/without fins"/4 -> Display4/1
  Gain/1 -> "Reactor, BaCl2/NH3, cylindrical, no walls, with algebraic loops, real gas in void volume, ideal gas in salt"/3

== system thermochemical/Reactors/Reactor, BaCl2//NH3, with algebraic loops, real gas in void volume, ideal gas in salt/Reactor, BaCl2//NH3, cylindrical, no walls, with algebraic loops, real gas in void volume, ideal gas in salt ==
  In3 : Inport
  In2 : Inport  Port=2
  In4 : Inport  Port=3
  "Reactor, BaCl2/NH3, no walls, with algebraic loops, real gas in void volume, ideal gas in salt" : thermochemical/Reactors/Reactor, BaCl2//NH3, with algebraic loops, real gas in void volume, ideal gas in salt/Reactor, BaCl2//NH3, no walls, with algebraic loops, real gas in void volume, ideal gas in salt  pairName=Barium chloride/Ammonia (BaCl2/NH3)  gasName=Ammonia gas (NH3)  binderName=ENG  N_salt=N_salt  N_binder=N_binder  K_cin=K_cin  V_void=V_void  fluid=fluid  Tr_init=Tr_init  X_init=X_init  N_gas_free_volume_init=N_gas_free_volume_init  m_composite_kg=4.162  m_salt_kg=3.1215  m_binder_kg=1.0405  m_gas_when_reactor_fully_charged=2.0424  T_ref=300  u_gas_at_T_ref=0  U_binder_at_T_ref=0  U_salt_at_X0_T_ref=0  cP_gas=42.5775  nu=8  cP_s0=75.1  Pr_0=1e-05  dh_r_0=38250  ds_r_0=232.38  M_binder=0.012011  cP_binder=714.36  P_dead_zone=0.0001  dn_dead_zone=0.0001  R=8.3145
      settings: SourceProductName=@ Thermochemical
  Out2 : Outport
  Out4 : Outport  Port=2
  Out3 : Outport  Port=3
  Out5 : Outport  Port=4
  Out1 : Outport  Port=5
  wires:
  In3/1 -> "Reactor, BaCl2/NH3, no walls, with algebraic loops, real gas in void volume, ideal gas in salt"/1  "dn/dt gas (mol/sec) > 0: gas in   < 0: gas out"
  In2/1 -> "Reactor, BaCl2/NH3, no walls, with algebraic loops, real gas in void volume, ideal gas in salt"/2  "enthalpy in (J/mol) (only needed if dn/dt gas > 0)"
  In4/1 -> "Reactor, BaCl2/NH3, no walls, with algebraic loops, real gas in void volume, ideal gas in salt"/3  "q out → in (W)"
  "Reactor, BaCl2/NH3, no walls, with algebraic loops, real gas in void volume, ideal gas in salt"/5 -> Out1/1  "X (0..1)"
  "Reactor, BaCl2/NH3, no walls, with algebraic loops, real gas in void volume, ideal gas in salt"/4 -> Out5/1  "Reaction phase"
  "Reactor, BaCl2/NH3, no walls, with algebraic loops, real gas in void volume, ideal gas in salt"/3 -> Out3/1  "h gas (void space) (J/mol)"
  "Reactor, BaCl2/NH3, no walls, with algebraic loops, real gas in void volume, ideal gas in salt"/2 -> Out4/1  "Pr (bar)"
  "Reactor, BaCl2/NH3, no walls, with algebraic loops, real gas in void volume, ideal gas in salt"/1 -> Out2/1  "Tr (K)"

== system thermochemical/Reactors/Reactor, BaCl2//NH3, with algebraic loops, real gas in void volume, ideal gas in salt/Reactor, BaCl2//NH3, no walls, with algebraic loops, real gas in void volume, ideal gas in salt ==
  In3 : Inport
  In2 : Inport  Port=2
  In4 : Inport  Port=3
  Reactor (no walls) : Subsystem
  Out2 : Outport
  Out1 : Outport  Port=2
  Out5 : Outport  Port=3
  Out3 : Outport  Port=4
  Out4 : Outport  Port=5
  wires:
  Reactor (no walls)/1(T_reactor (K)) -> Out2/1  "Tr (K)"
  In4/1 -> Reactor (no walls)/1(q reactor → wall (W))  "q out → in (W)"
  In2/1 -> Reactor (no walls)/2(enthalpy_in (J/mol) (only if dn_gas > 0))  "enthalpy in (J/mol) (only needed if dn/dt gas > 0)"
  In3/1 -> Reactor (no walls)/3(dn_gas (mol/sec) (if > 0: gas in if < 0: gas out))  "dn/dt gas (mol/sec) > 0: gas in   < 0: gas out"
  Reactor (no walls)/2(X (0..1)) -> Out4/1  "X (0..1)"
  Reactor (no walls)/3(Reactor phase) -> Out3/1  "Reaction phase"
  Reactor (no walls)/4(h_reactor_free_volume (J/mol)) -> Out5/1  "h gas void space (J/mol)"
  Reactor (no walls)/5(P_reactor (bar)) -> Out1/1  "Pr (bar)"

== system thermochemical/Reactors/Reactor, BaCl2//NH3, with algebraic loops, real gas in void volume, real gas in salt/Reactor, BaCl2, cylindrical, finned tube, with algebraic loops, real gas in void volume, real gas in salt ==
  In3 : Inport
  In1 : Inport  Port=2
  In2 : Inport  Port=3
  In4 : Inport  Port=4
  Display4 : Display
  Gain : Gain  Gain=-1
  "Reactor, BaCl2/NH3, cylindrical, no walls, with algebraic loops, real gas in void volume, real gas in salt" : thermochemical/Reactors/Reactor, BaCl2//NH3, with algebraic loops, real gas in void volume, real gas in salt/Reactor, BaCl2//NH3, cylindrical, no walls, with algebraic loops, real gas in void volume, real gas in salt  pairName=Barium chloride/Ammonia (BaCl2/NH3)  gasName=Ammonia gas (NH3)  binderName=ENG  tao_salt=0.75  rho_composite=300  K_cin=1e-3  fluid=nh3_v3  Lr=1.5  Lr_total=1.6  Dr=0.11  Ddiff=0.018  Tr_init=300  X_init=0.1  Vr_L=15.2053  m_composite_kg=4.162  m_salt_kg=3.1215  m_binder_kg=1.0405  m_gas_when_reactor_fully_charged_kg=2.0423  kWh_cold=0.77838  N_salt=14.9906  N_binder=86.6307  V_void=0.001332  N_gas_free_volume_init=0.16063
      settings: SourceProductName=@ Thermochemical
  "Wall, tube with/without fins" : thermochemical/Walls/Wall, tube with//without fins  L_m=1.6  OD_mm=114  e_mm=2  material_tube=Stainless steel AISI316  cp_tube=490.8  rho_tube=8023  height_fin_mm=0  thickness_fin_mm=0  pitch_fin_mm=0  material_fin=Steel  cp_fin=464.5  rho_fin=7847  lambda_fin=64.65  Tinit=300  mass_tube=4.5571  mass_fin=0  mass_total=4.5571  s_inner=0.56297  s_outer=0.57303
      settings: SourceProductName=@ Thermochemical
  composite-wall contact heat transfer coefficient (W/m2/K) : Constant  Value=300
  Out3 : Outport
  Out2 : Outport  Port=2
  Out4 : Outport  Port=3
  Out1 : Outport  Port=4
  Out5 : Outport  Port=5
  Out6 : Outport  Port=6
  Out7 : Outport  Port=7
  Out8 : Outport  Port=8
  wires:
  In4/1 -> "Reactor, BaCl2/NH3, cylindrical, no walls, with algebraic loops, real gas in void volume, real gas in salt"/2  "enthalpy in (J/mol) (only needed if dn/dt gas > 0)"
  In2/1 -> "Reactor, BaCl2/NH3, cylindrical, no walls, with algebraic loops, real gas in void volume, real gas in salt"/1  "dn/dt gas (mol/sec) > 0: gas in   < 0: gas out"
  "Wall, tube with/without fins"/1 -> Out3/1  "T wall (K)"
  "Reactor, BaCl2/NH3, cylindrical, no walls, with algebraic loops, real gas in void volume, real gas in salt"/2 -> Out4/1  "Pr (bar)"
  "Reactor, BaCl2/NH3, cylindrical, no walls, with algebraic loops, real gas in void volume, real gas in salt"/5 -> Out6/1  "X (0..1)"
  In1/1 -> "Wall, tube with/without fins"/2  "h outer (W/m2/K)"
  "Wall, tube with/without fins"/3 -> Out8/1  "Q wall → outer (W)"
  In3/1 -> "Wall, tube with/without fins"/1  "T outer (K)"
  "Reactor, BaCl2/NH3, cylindrical, no walls, with algebraic loops, real gas in void volume, real gas in salt"/3 -> Out1/1  "h gas (void space) (J/mol)"
  composite-wall contact heat transfer coefficient (W/m2/K)/1 -> "Wall, tube with/without fins"/4
  "Wall, tube with/without fins"/2 -> Out7/1, Gain/1  "Q inner → wall (W)"
  "Reactor, BaCl2/NH3, cylindrical, no walls, with algebraic loops, real gas in void volume, real gas in salt"/4 -> Out5/1  "Reaction phase"
  "Reactor, BaCl2/NH3, cylindrical, no walls, with algebraic loops, real gas in void volume, real gas in salt"/1 -> "Wall, tube with/without fins"/3, Out2/1  "Tr (K)"
  "Wall, tube with/without fins"/4 -> Display4/1
  Gain/1 -> "Reactor, BaCl2/NH3, cylindrical, no walls, with algebraic loops, real gas in void volume, real gas in salt"/3

== system thermochemical/Reactors/Reactor, BaCl2//NH3, with algebraic loops, real gas in void volume, real gas in salt/Reactor, BaCl2//NH3, cylindrical, no walls, with algebraic loops, real gas in void volume, real gas in salt ==
  In3 : Inport
  In2 : Inport  Port=2
  In4 : Inport  Port=3
  "Reactor, BaCl2/NH3, no walls, with algebraic loops, real gas in void volume, real gas in salt" : thermochemical/Reactors/Reactor, BaCl2//NH3, with algebraic loops, real gas in void volume, real gas in salt/Reactor, BaCl2//NH3, no walls, with algebraic loops, real gas in void volume, real gas in salt  pairName=Barium chloride/Ammonia (BaCl2/NH3)  gasName=Ammonia gas (NH3)  binderName=ENG  N_salt=N_salt  N_binder=N_binder  K_cin=K_cin  V_void=V_void  fluid=fluid  Tr_init=Tr_init  X_init=X_init  N_gas_free_volume_init=N_gas_free_volume_init  m_composite_kg=4.1639  m_salt_kg=3.1235  m_binder_kg=1.0405  m_gas_when_reactor_fully_charged=2.0436  T_ref=300  u_gas_at_T_ref=0  U_binder_at_T_ref=0  U_salt_at_X0_T_ref=0  cP_gas=42.5775  nu=8  cP_s0=75.1  Pr_0=1e-05  dh_r_0=38250  ds_r_0=232.38  M_binder=0.012011  cP_binder=714.36  P_dead_zone=0.0001  dn_dead_zone=0.0001  R=8.3145
      settings: SourceProductName=@ Thermochemical
  Out2 : Outport
  Out4 : Outport  Port=2
  Out3 : Outport  Port=3
  Out5 : Outport  Port=4
  Out1 : Outport  Port=5
  wires:
  In3/1 -> "Reactor, BaCl2/NH3, no walls, with algebraic loops, real gas in void volume, real gas in salt"/1  "dn/dt gas (mol/sec) > 0: gas in   < 0: gas out"
  In2/1 -> "Reactor, BaCl2/NH3, no walls, with algebraic loops, real gas in void volume, real gas in salt"/2  "enthalpy in (J/mol) (only needed if dn/dt gas > 0)"
  In4/1 -> "Reactor, BaCl2/NH3, no walls, with algebraic loops, real gas in void volume, real gas in salt"/3  "q out → in (W)"
  "Reactor, BaCl2/NH3, no walls, with algebraic loops, real gas in void volume, real gas in salt"/5 -> Out1/1  "X (0..1)"
  "Reactor, BaCl2/NH3, no walls, with algebraic loops, real gas in void volume, real gas in salt"/4 -> Out5/1  "Reaction phase"
  "Reactor, BaCl2/NH3, no walls, with algebraic loops, real gas in void volume, real gas in salt"/3 -> Out3/1  "h gas (void space) (J/mol)"
  "Reactor, BaCl2/NH3, no walls, with algebraic loops, real gas in void volume, real gas in salt"/2 -> Out4/1  "Pr (bar)"
  "Reactor, BaCl2/NH3, no walls, with algebraic loops, real gas in void volume, real gas in salt"/1 -> Out2/1  "Tr (K)"

== system thermochemical/Reactors/Reactor, BaCl2//NH3, with algebraic loops, real gas in void volume, real gas in salt/Reactor, BaCl2//NH3, no walls, with algebraic loops, real gas in void volume, real gas in salt ==
  In3 : Inport
  In2 : Inport  Port=2
  In4 : Inport  Port=3
  Reactor (no walls) : Subsystem
  Out2 : Outport
  Out1 : Outport  Port=2
  Out5 : Outport  Port=3
  Out3 : Outport  Port=4
  Out4 : Outport  Port=5
  wires:
  Reactor (no walls)/5(P_reactor (bar)) -> Out1/1  "Pr (bar)"
  Reactor (no walls)/4(h_reactor_free_volume (J/mol)) -> Out5/1  "h gas void space (J/mol)"
  Reactor (no walls)/3(Reactor phase) -> Out3/1  "Reaction phase"
  Reactor (no walls)/2(X (0..1)) -> Out4/1  "X (0..1)"
  In3/1 -> Reactor (no walls)/3(dn_gas (mol/sec) (if > 0: gas in if < 0: gas out))  "dn/dt gas (mol/sec) > 0: gas in   < 0: gas out"
  In2/1 -> Reactor (no walls)/2(enthalpy_in (J/mol) (only if dn_gas > 0))  "enthalpy in (J/mol) (only needed if dn/dt gas > 0)"
  In4/1 -> Reactor (no walls)/1(q reactor → wall (W))  "q out → in (W)"
  Reactor (no walls)/1(T_reactor (K)) -> Out2/1  "Tr (K)"

== system thermochemical/Thermodynamic fluid properties/Thermodynamic property (non-saturated)/Subsystem1 ==
  In1 : Inport
  In2 : Inport  Port=2
  Constant : Constant  Value=str2num(reciprocVar)
  Math Function : Math  Operator=reciprocal  SaturateOnIntegerOverflow=on
  look-up table 2D : Lookup_n-D  BreakpointsForDimension1=lookup2D_BreakPoint1  BreakpointsForDimension2=lookup2D_BreakPoint2  BreakpointsForDimension3=[5, 7]  BeginIndexSearchUsingPreviousIndexResult=on  Table=lookup2D_Data  ExtrapMethod=Clip  InternalRulePriority=Speed  RndMeth=Simplest  InputSameDT=on
  switch2 : Switch  Criteria=u2 > Threshold
  Out1 : Outport
  wires:
  In2/1 -> look-up table 2D/2
  switch2/1 -> Out1/1
  Constant/1 -> switch2/2
  In1/1 -> look-up table 2D/1
  look-up table 2D/1 -> Math Function/1, switch2/3
  Math Function/1 -> switch2/1
